simulink model "GP_DS"  (R2018b)
settings: Solver=ode5  StartTime=0.0  StopTime=N*Tb  FixedStep=Tsampling  RelTol=1e-3
values from neighbouring files (symbols this model uses):
  Eb = 2    [GP_DS_Script.m]
  fp = 2*Rc    (= 20000)    [GP_DS_Script.m]
  Tb = 1/Rb    (= 0.001)    [GP_DS_Script.m]
  Tc = 1/Rc    (= 0.0001)    [GP_DS_Script.m]
  Tsampling = Tc/100    (= 1e-06)    [GP_DS_Script.m]
libraries: commrandsrc3 x1, commseqgen3 x1, commdigbbndpm3 x1, commutil2 x1
settings Model: Creator=lukit  LastModifiedBy=lukit

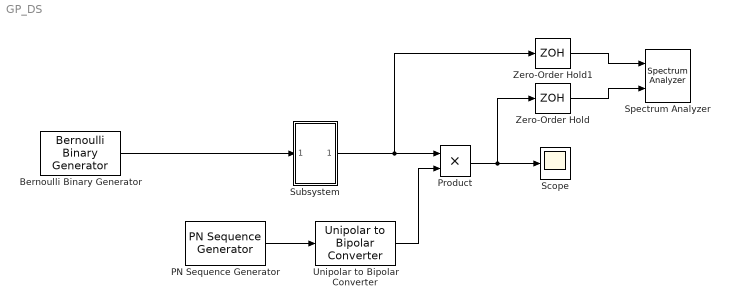
== system GP_DS ==
  Bernoulli Binary Generator : commrandsrc3/Bernoulli Binary Generator  ProbabilityOfZero=0.5  SeedSource=Auto  Seed=0  SampleTime=Tb  SamplesPerFrame=1  OutputDataType=double  SimulateUsing=Interpreted execution
  PN Sequence Generator : commseqgen3/PN Sequence Generator  poly=[5,2,0]  ini_sta=[0,0,0,0,1]  outBitMaskSource=Dialog parameter  shift=0  outVarSiz=off  maxOutSizeMode=Dialog parameter  maxOutSize=[10 1]  Ts=Tc  sampPerFrame=1  reset=off  bitPackedOutputs=off  outDataType=double  numPackedBits=8  bitPackDataSigned=off  bitPackedOutDType=double
      settings: SourceProductName=Communications System Toolbox
  Product : Product
  Scope : Scope
  Spectrum Analyzer : SpectrumAnalyzer  NumInputPorts=2
  Subsystem : Subsystem
  Unipolar to Bipolar Converter : commutil2/Unipolar to Bipolar Converter  M=2  polarity=Positive  dataType=Inherit via internal rule
      settings: SourceProductName=Communications System Toolbox
  Zero-Order Hold : ZeroOrderHold  SampleTime=-1
  Zero-Order Hold1 : ZeroOrderHold  SampleTime=-1
  wires:
  Bernoulli Binary Generator/1 -> Subsystem/1(In1)
  PN Sequence Generator/1 -> Unipolar to Bipolar Converter/1
  Subsystem/1(Out1) -> Zero-Order Hold1/1, Product/1
  Unipolar to Bipolar Converter/1 -> Product/2
  Product/1 -> Zero-Order Hold/1, Scope/1
  Zero-Order Hold/1 -> Spectrum Analyzer/2
  Zero-Order Hold1/1 -> Spectrum Analyzer/1

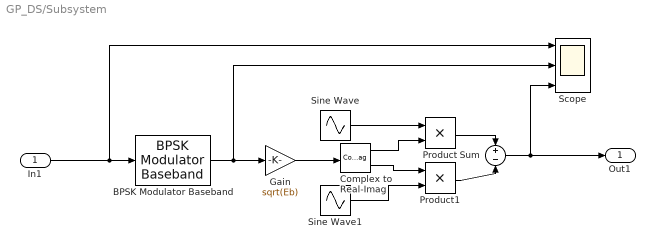
== system GP_DS/Subsystem ==
  In1 : Inport
  BPSK Modulator Baseband : commdigbbndpm3/BPSK Modulator Baseband  Ph=0  outDtype=double  outWordLen=16  outUDDataType=sfix(16)  outFracLenMode=Best precision  outFracLen=15  outDataTypeStr=double  outLastDataTypeStr=double
  Complex to Real-Imag : ComplexToRealImag
  Gain : Gain  Gain=sqrt(Eb)
  Product : Product
  Product1 : Product
  Scope : Scope  NumInputPorts=3
  Sine Wave : Sin  Frequency=2*pi*fp  Phase=pi/2  SampleTime=Tsampling
  Sine Wave1 : Sin  Frequency=2*pi*fp  SampleTime=Tsampling
  Sum : Sum  Inputs=+-
  Out1 : Outport
  wires:
  In1/1 -> BPSK Modulator Baseband/1, Scope/1
  Complex to Real-Imag/2 -> Product1/1
  Product1/1 -> Sum/2
  Product/1 -> Sum/1
  Sine Wave1/1 -> Product1/2
  Sum/1 -> Out1/1, Scope/3
  Sine Wave/1 -> Product/1
  Gain/1 -> Complex to Real-Imag/1
  Complex to Real-Imag/1 -> Product/2
  BPSK Modulator Baseband/1 -> Gain/1, Scope/2
